simulink model "multiportswitch_bus_test"  (Simulink 8.4)
settings: Solver=VariableStepDiscrete  StartTime=0.0  StopTime=0  MaxStep=1  RelTol=1e-3
settings Model: Creator=arnaud  LastModifiedBy=arnaud
settings DataIOCC: SaveFormat=Structure  SignalLoggingSaveFormat=Dataset
settings OptimizationCC: ExpressionDepthLimit=128
settings DebuggingCC: UnderspecifiedInitializationDetection=Simplified  MergeDetectMultiDrivingBlocksExec=error  FcnCallInpInsideContextMsg=EnableAllAsError  StateNameClashWarn=none
settings GRTTargetCC: CombineOutputUpdateFcns=on  GRTInterface=off

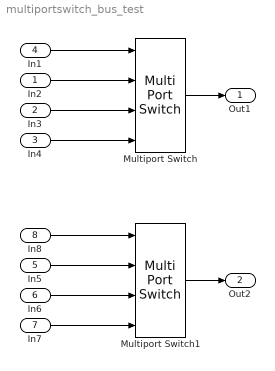
== system multiportswitch_bus_test ==
  In2 : Inport  OutDataTypeStr=Bus: BusA  PortDimensions=[2 3]  BusOutputAsStruct=on
  In3 : Inport  Port=2  OutDataTypeStr=Bus: BusA  PortDimensions=[2 3]  BusOutputAsStruct=on
  In4 : Inport  Port=3  OutDataTypeStr=Bus: BusA  PortDimensions=[2 3]  BusOutputAsStruct=on
  In1 : Inport  Port=4  OutDataTypeStr=int8  PortDimensions=[2 3]
  In5 : Inport  Port=5  OutDataTypeStr=Bus: BusB  PortDimensions=1  BusOutputAsStruct=on
  In6 : Inport  Port=6  OutDataTypeStr=Bus: BusB  PortDimensions=1  BusOutputAsStruct=on
  In7 : Inport  Port=7  OutDataTypeStr=Bus: BusB  PortDimensions=1  BusOutputAsStruct=on
  In8 : Inport  Port=8  OutDataTypeStr=int8  PortDimensions=1
  Multiport Switch : MultiPortSwitch  DataPortOrder=Specify indices  DataPortIndices={0,[2,3]}  DataPortForDefault=Additional data port  DiagnosticForDefault=Warning
  Multiport Switch1 : MultiPortSwitch  DataPortOrder=Zero-based contiguous  Inputs=2  DataPortIndices={1,[2,3]}  DataPortForDefault=Additional data port  DiagnosticForDefault=Warning
  Out1 : Outport
  Out2 : Outport  Port=2
  wires:
  Multiport Switch/1 -> Out1/1
  In2/1 -> Multiport Switch/2
  In3/1 -> Multiport Switch/3
  In4/1 -> Multiport Switch/4
  In1/1 -> Multiport Switch/1
  Multiport Switch1/1 -> Out2/1
  In5/1 -> Multiport Switch1/2
  In6/1 -> Multiport Switch1/3
  In7/1 -> Multiport Switch1/4
  In8/1 -> Multiport Switch1/1
